simulink model "Joint_space_Traj"  (R2019b)
settings: Solver=FixedStepAuto  StartTime=0.0  StopTime=8  FixedStep=0.01  RelTol=1e-3
settings Model: Creator=gasserelazab  LastModifiedBy=gasserelazab

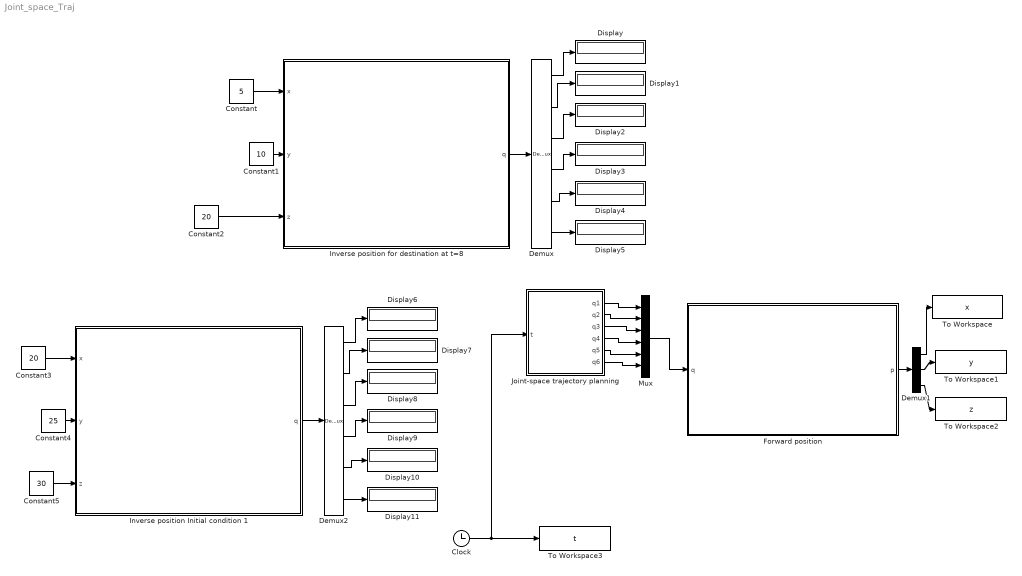
== system Joint_space_Traj ==
  Clock : Clock
  Constant : Constant  Value=5
  Constant1 : Constant  Value=10
  Constant2 : Constant  Value=20
  Constant3 : Constant  Value=20
  Constant4 : Constant  Value=25
  Constant5 : Constant  Value=30
  Demux : Demux  Outputs=6
  Demux1 : Demux  Outputs=3
  Demux2 : Demux  Outputs=6
  Display{,1..11} (12 alike) : Display
  "Forward position " : MATLAB Function  TreatAsAtomicUnit=on
  Inverse position Initial condition 1 : MATLAB Function  TreatAsAtomicUnit=on
  "Inverse position for destination at t=8 " : MATLAB Function  TreatAsAtomicUnit=on
  "Joint-space trajectory planning " : MATLAB Function  TreatAsAtomicUnit=on
  Mux : Mux  Inputs=6
  To Workspace : ToWorkspace  VariableName=x  SampleTime=-1
  To Workspace1 : ToWorkspace  VariableName=y  SampleTime=-1
  To Workspace2 : ToWorkspace  VariableName=z  SampleTime=-1
  To Workspace3 : ToWorkspace  VariableName=t  SampleTime=-1
  wires:
  Constant2/1 -> "Inverse position for destination at t=8 "/3(z)
  Constant1/1 -> "Inverse position for destination at t=8 "/2(y)
  Constant/1 -> "Inverse position for destination at t=8 "/1(x)
  "Inverse position for destination at t=8 "/1(q) -> Demux/1
  Demux/1 -> Display/1
  Demux/2 -> Display1/1
  Demux/3 -> Display2/1
  Demux/4 -> Display3/1
  Demux/5 -> Display4/1
  Demux/6 -> Display5/1
  Clock/1 -> To Workspace3/1, "Joint-space trajectory planning "/1(t)
  "Joint-space trajectory planning "/1(q1) -> Mux/1
  "Joint-space trajectory planning "/2(q2) -> Mux/2
  "Joint-space trajectory planning "/3(q3) -> Mux/3
  "Joint-space trajectory planning "/4(q4) -> Mux/4
  "Joint-space trajectory planning "/5(q5) -> Mux/5
  "Joint-space trajectory planning "/6(q6) -> Mux/6
  Mux/1 -> "Forward position "/1(q)
  "Forward position "/1(p) -> Demux1/1
  Demux1/1 -> To Workspace/1
  Demux1/2 -> To Workspace1/1
  Demux1/3 -> To Workspace2/1
  Demux2/4 -> Display9/1
  Inverse position Initial condition 1/1(q) -> Demux2/1
  Demux2/5 -> Display10/1
  Demux2/6 -> Display11/1
  Demux2/3 -> Display8/1
  Demux2/2 -> Display7/1
  Constant4/1 -> Inverse position Initial condition 1/2(y)
  Constant5/1 -> Inverse position Initial condition 1/3(z)
  Demux2/1 -> Display6/1
  Constant3/1 -> Inverse position Initial condition 1/1(x)

== matlab function Joint_space_Traj/Inverse position for destination at t=8  ==
  data: q output; x input; y input; z input
function q   = fcn(x, y, z)

qnew=[0;0;0;0;0;0];
qold=[50;50;50;50;50;50];

i=100;
dog=true;

while (i>0 && dog)
    q1=qold(1,1);
    q2=qold(2,1);
    q3=qold(3,1);
    q4=qold(4,1);
    q5=qold(5,1);
    q6=qold(6,1);
    
    F= [ 10*cos((pi*(q1 - 90))/180)*sin((pi*(q2 - 90))/180) - 10*sin((pi*(q5 + 90))/180)*(sin((pi*(q1 - 90))/180)*sin((pi*(q4 + 90))/180) - cos((pi*(q1 - 90))/180)*cos((pi*(q2 - 90))/180)*cos((pi*(q4 + 90))/180)) - x + cos((pi*(q1 - 90))/180)*sin((pi*(q2 - 90))/180)*(q3 + 10) - 10*cos((pi*(q1 - 90))/180)*cos((pi*(q5 + 90))/180)*sin((pi*(q2 - 90))/180);...
 10*sin((pi*(q5 + 90))/180)*(cos((pi*(q1 - 90))/180)*sin((pi*(q4 + 90))/180) + cos((pi*(q2 - 90))/180)*cos((pi*(q4 + 90))/180)*sin((pi*(q1 - 90))/180)) - y + 10*sin((pi*(q1 - 90))/180)*sin((pi*(q2 - 90))/180) + sin((pi*(q1 - 90))/180)*sin((pi*(q2 - 90))/180)*(q3 + 10) - 10*cos((pi*(q5 + 90))/180)*sin((pi*(q1 - 90))/180)*sin((pi*(q2 - 90))/180);...
                                                                                                                                                10*cos((pi*(q2 - 90))/180) - z + cos((pi*(q2 - 90))/180)*(q3 + 10) - 10*cos((pi*(q2 - 90))/180)*cos((pi*(q5 + 90))/180) - 10*cos((pi*(q4 + 90))/180)*sin((pi*(q2 - 90))/180)*sin((pi*(q5 + 90))/180) + 10];
 FJ= [ (pi*cos((pi*(q5 + 90))/180)*sin((pi*(q1 - 90))/180)*sin((pi*(q2 - 90))/180))/18 - (pi*sin((pi*(q1 - 90))/180)*sin((pi*(q2 - 90))/180))/18 - (pi*sin((pi*(q1 - 90))/180)*sin((pi*(q2 - 90))/180)*(q3 + 10))/180 - 10*sin((pi*(q5 + 90))/180)*((pi*cos((pi*(q1 - 90))/180)*sin((pi*(q4 + 90))/180))/180 + (pi*cos((pi*(q2 - 90))/180)*cos((pi*(q4 + 90))/180)*sin((pi*(q1 - 90))/180))/180), (pi*cos((pi*(q1 - 90))/180)*cos((pi*(q2 - 90))/180))/18 + (pi*cos((pi*(q1 - 90))/180)*cos((pi*(q2 - 90))/180)*(q3 + 10))/180 - (pi*cos((pi*(q1 - 90))/180)*cos((pi*(q2 - 90))/180)*cos((pi*(q5 + 90))/180))/18 - (pi*cos((pi*(q1 - 90))/180)*cos((pi*(q4 + 90))/180)*sin((pi*(q2 - 90))/180)*sin((pi*(q5 + 90))/180))/18, cos((pi*(q1 - 90))/180)*sin((pi*(q2 - 90))/180), -10*sin((pi*(q5 + 90))/180)*((pi*cos((pi*(q4 + 90))/180)*sin((pi*(q1 - 90))/180))/180 + (pi*cos((pi*(q1 - 90))/180)*cos((pi*(q2 - 90))/180)*sin((pi*(q4 + 90))/180))/180), (pi*cos((pi*(q1 - 90))/180)*sin((pi*(q2 - 90))/180)*sin((pi*(q5 + 90))/180))/18 - (pi*cos((pi*(q5 + 90))/180)*(sin((pi*(q1 - 90))/180)*sin((pi*(q4 + 90))/180) - cos((pi*(q1 - 90))/180)*cos((pi*(q2 - 90))/180)*cos((pi*(q4 + 90))/180)))/18, 0;...
 (pi*cos((pi*(q1 - 90))/180)*sin((pi*(q2 - 90))/180))/18 - 10*sin((pi*(q5 + 90))/180)*((pi*sin((pi*(q1 - 90))/180)*sin((pi*(q4 + 90))/180))/180 - (pi*cos((pi*(q1 - 90))/180)*cos((pi*(q2 - 90))/180)*cos((pi*(q4 + 90))/180))/180) + (pi*cos((pi*(q1 - 90))/180)*sin((pi*(q2 - 90))/180)*(q3 + 10))/180 - (pi*cos((pi*(q1 - 90))/180)*cos((pi*(q5 + 90))/180)*sin((pi*(q2 - 90))/180))/18, (pi*cos((pi*(q2 - 90))/180)*sin((pi*(q1 - 90))/180))/18 + (pi*cos((pi*(q2 - 90))/180)*sin((pi*(q1 - 90))/180)*(q3 + 10))/180 - (pi*cos((pi*(q2 - 90))/180)*cos((pi*(q5 + 90))/180)*sin((pi*(q1 - 90))/180))/18 - (pi*cos((pi*(q4 + 90))/180)*sin((pi*(q1 - 90))/180)*sin((pi*(q2 - 90))/180)*sin((pi*(q5 + 90))/180))/18, sin((pi*(q1 - 90))/180)*sin((pi*(q2 - 90))/180),  10*sin((pi*(q5 + 90))/180)*((pi*cos((pi*(q1 - 90))/180)*cos((pi*(q4 + 90))/180))/180 - (pi*cos((pi*(q2 - 90))/180)*sin((pi*(q1 - 90))/180)*sin((pi*(q4 + 90))/180))/180), (pi*cos((pi*(q5 + 90))/180)*(cos((pi*(q1 - 90))/180)*sin((pi*(q4 + 90))/180) + cos((pi*(q2 - 90))/180)*cos((pi*(q4 + 90))/180)*sin((pi*(q1 - 90))/180)))/18 + (pi*sin((pi*(q1 - 90))/180)*sin((pi*(q2 - 90))/180)*sin((pi*(q5 + 90))/180))/18, 0;...
                                                                                                                                                                                                                                                                                                                                                                                         0,                                                                                                 (pi*cos((pi*(q5 + 90))/180)*sin((pi*(q2 - 90))/180))/18 - (pi*sin((pi*(q2 - 90))/180)*(q3 + 10))/180 - (pi*sin((pi*(q2 - 90))/180))/18 - (pi*cos((pi*(q2 - 90))/180)*cos((pi*(q4 + 90))/180)*sin((pi*(q5 + 90))/180))/18,                         cos((pi*(q2 - 90))/180),                                                                                           (pi*sin((pi*(q2 - 90))/180)*sin((pi*(q4 + 90))/180)*sin((pi*(q5 + 90))/180))/18,                                                                                                     (pi*cos((pi*(q2 - 90))/180)*sin((pi*(q5 + 90))/180))/18 - (pi*cos((pi*(q4 + 90))/180)*cos((pi*(q5 + 90))/180)*sin((pi*(q2 - 90))/180))/18, 0];
 

    inverseFJ= transpose(FJ)*(inv(FJ*transpose(FJ)));
        
 
    qnew=qold-inverseFJ*F;
    %disp(inverseFJ*F);
    
  
   
    count=0;
   
   	for xx = 1:6
        if  ((qnew(xx,1)-qold(xx,1)<0.1) && (qnew(xx,1)-qold(xx,1)>-0.1 ))       
             count=count+1;
         end
   
    end
    
    if( count == 6)
        dog=false;
    end
    
    i=i-1;
    
    %disp(i);
    
    qold=qnew;
    
end
q=qold;

== matlab function Joint_space_Traj/Joint-space trajectory planning  ==
  data: t input; q1 output; q2 output; q3 output; q4 output; q5 output; q6 output
function [q1,q2,q3,q4,q5,q6] = fcn(t)

q1= -21.89 + 1.75125*t^(2) - 0.146*t^(3);
q2= 38.51 + 1.415*t^(2) -0.118*t^(3);
q3= 14.89 + -1.30125*t^(2) + 0.1084375*t^(3);
q4= 20.75 + 0.3740526*t^(2) - 0.031171875*t^(3);
q5= 8.891 + 1.0542*t^(2) - 0.0878*t^(3);
q6=0;

== matlab function Joint_space_Traj/Forward position  ==
  data: p output; q input
function p  = fcn(q)
q1= q(1);
q2= q(2);
q3= q(3);
q4= q(4);
q5= q(5);
q6= q(6);
L1=10;
L2=10;
L3=10;
L4=10;
pp= [ sin((pi*q6)/180)*(cos((pi*(q4 + 90))/180)*sin((pi*(q1 - 90))/180) + cos((pi*(q1 - 90))/180)*cos((pi*(q2 - 90))/180)*sin((pi*(q4 + 90))/180)) - cos((pi*q6)/180)*(cos((pi*(q5 + 90))/180)*(sin((pi*(q1 - 90))/180)*sin((pi*(q4 + 90))/180) - cos((pi*(q1 - 90))/180)*cos((pi*(q2 - 90))/180)*cos((pi*(q4 + 90))/180)) - cos((pi*(q1 - 90))/180)*sin((pi*(q2 - 90))/180)*sin((pi*(q5 + 90))/180)),   sin((pi*q6)/180)*(cos((pi*(q5 + 90))/180)*(sin((pi*(q1 - 90))/180)*sin((pi*(q4 + 90))/180) - cos((pi*(q1 - 90))/180)*cos((pi*(q2 - 90))/180)*cos((pi*(q4 + 90))/180)) - cos((pi*(q1 - 90))/180)*sin((pi*(q2 - 90))/180)*sin((pi*(q5 + 90))/180)) + cos((pi*q6)/180)*(cos((pi*(q4 + 90))/180)*sin((pi*(q1 - 90))/180) + cos((pi*(q1 - 90))/180)*cos((pi*(q2 - 90))/180)*sin((pi*(q4 + 90))/180)), - sin((pi*(q5 + 90))/180)*(sin((pi*(q1 - 90))/180)*sin((pi*(q4 + 90))/180) - cos((pi*(q1 - 90))/180)*cos((pi*(q2 - 90))/180)*cos((pi*(q4 + 90))/180)) - cos((pi*(q1 - 90))/180)*cos((pi*(q5 + 90))/180)*sin((pi*(q2 - 90))/180), cos((pi*(q1 - 90))/180)*sin((pi*(q2 - 90))/180)*(L2 + q3) - L4*(sin((pi*(q5 + 90))/180)*(sin((pi*(q1 - 90))/180)*sin((pi*(q4 + 90))/180) - cos((pi*(q1 - 90))/180)*cos((pi*(q2 - 90))/180)*cos((pi*(q4 + 90))/180)) + cos((pi*(q1 - 90))/180)*cos((pi*(q5 + 90))/180)*sin((pi*(q2 - 90))/180)) + L3*cos((pi*(q1 - 90))/180)*sin((pi*(q2 - 90))/180);
 cos((pi*q6)/180)*(cos((pi*(q5 + 90))/180)*(cos((pi*(q1 - 90))/180)*sin((pi*(q4 + 90))/180) + cos((pi*(q2 - 90))/180)*cos((pi*(q4 + 90))/180)*sin((pi*(q1 - 90))/180)) + sin((pi*(q1 - 90))/180)*sin((pi*(q2 - 90))/180)*sin((pi*(q5 + 90))/180)) - sin((pi*q6)/180)*(cos((pi*(q1 - 90))/180)*cos((pi*(q4 + 90))/180) - cos((pi*(q2 - 90))/180)*sin((pi*(q1 - 90))/180)*sin((pi*(q4 + 90))/180)), - sin((pi*q6)/180)*(cos((pi*(q5 + 90))/180)*(cos((pi*(q1 - 90))/180)*sin((pi*(q4 + 90))/180) + cos((pi*(q2 - 90))/180)*cos((pi*(q4 + 90))/180)*sin((pi*(q1 - 90))/180)) + sin((pi*(q1 - 90))/180)*sin((pi*(q2 - 90))/180)*sin((pi*(q5 + 90))/180)) - cos((pi*q6)/180)*(cos((pi*(q1 - 90))/180)*cos((pi*(q4 + 90))/180) - cos((pi*(q2 - 90))/180)*sin((pi*(q1 - 90))/180)*sin((pi*(q4 + 90))/180)),   sin((pi*(q5 + 90))/180)*(cos((pi*(q1 - 90))/180)*sin((pi*(q4 + 90))/180) + cos((pi*(q2 - 90))/180)*cos((pi*(q4 + 90))/180)*sin((pi*(q1 - 90))/180)) - cos((pi*(q5 + 90))/180)*sin((pi*(q1 - 90))/180)*sin((pi*(q2 - 90))/180), L4*(sin((pi*(q5 + 90))/180)*(cos((pi*(q1 - 90))/180)*sin((pi*(q4 + 90))/180) + cos((pi*(q2 - 90))/180)*cos((pi*(q4 + 90))/180)*sin((pi*(q1 - 90))/180)) - cos((pi*(q5 + 90))/180)*sin((pi*(q1 - 90))/180)*sin((pi*(q2 - 90))/180)) + sin((pi*(q1 - 90))/180)*sin((pi*(q2 - 90))/180)*(L2 + q3) + L3*sin((pi*(q1 - 90))/180)*sin((pi*(q2 - 90))/180);
                                                                                                                                                                                 cos((pi*q6)/180)*(cos((pi*(q2 - 90))/180)*sin((pi*(q5 + 90))/180) - cos((pi*(q4 + 90))/180)*cos((pi*(q5 + 90))/180)*sin((pi*(q2 - 90))/180)) - sin((pi*q6)/180)*sin((pi*(q2 - 90))/180)*sin((pi*(q4 + 90))/180),                                                                                                                                                                                 - sin((pi*q6)/180)*(cos((pi*(q2 - 90))/180)*sin((pi*(q5 + 90))/180) - cos((pi*(q4 + 90))/180)*cos((pi*(q5 + 90))/180)*sin((pi*(q2 - 90))/180)) - cos((pi*q6)/180)*sin((pi*(q2 - 90))/180)*sin((pi*(q4 + 90))/180),                                                                                                     - cos((pi*(q2 - 90))/180)*cos((pi*(q5 + 90))/180) - cos((pi*(q4 + 90))/180)*sin((pi*(q2 - 90))/180)*sin((pi*(q5 + 90))/180),                                                                                                                                                L1 - L4*(cos((pi*(q2 - 90))/180)*cos((pi*(q5 + 90))/180) + cos((pi*(q4 + 90))/180)*sin((pi*(q2 - 90))/180)*sin((pi*(q5 + 90))/180)) + cos((pi*(q2 - 90))/180)*(L2 + q3) + L3*cos((pi*(q2 - 90))/180);
                                                                                                                                                                                                                                                                                                                                                                                               0,                                                                                                                                                                                                                                                                                                                                                                                                 0,                                                                                                                                                                                                                               0,                                                                                                                                                                                                                                                                                                                                                   1];
x=pp(1,4);
y=pp(2,4);
z=pp(3,4);
p= [x;y;z];

== matlab function Joint_space_Traj/Inverse position Initial condition 1 ==
  data: q output; x input; y input; z input
function q   = fcn(x, y, z)

qnew=[0;0;0;0;0;0];
qold=[50;50;50;50;50;50];

i=100;
dog=true;

while (i>0 && dog)
    q1=qold(1,1);
    q2=qold(2,1);
    q3=qold(3,1);
    q4=qold(4,1);
    q5=qold(5,1);
    q6=qold(6,1);
    
    F= [ 10*cos((pi*(q1 - 90))/180)*sin((pi*(q2 - 90))/180) - 10*sin((pi*(q5 + 90))/180)*(sin((pi*(q1 - 90))/180)*sin((pi*(q4 + 90))/180) - cos((pi*(q1 - 90))/180)*cos((pi*(q2 - 90))/180)*cos((pi*(q4 + 90))/180)) - x + cos((pi*(q1 - 90))/180)*sin((pi*(q2 - 90))/180)*(q3 + 10) - 10*cos((pi*(q1 - 90))/180)*cos((pi*(q5 + 90))/180)*sin((pi*(q2 - 90))/180);...
 10*sin((pi*(q5 + 90))/180)*(cos((pi*(q1 - 90))/180)*sin((pi*(q4 + 90))/180) + cos((pi*(q2 - 90))/180)*cos((pi*(q4 + 90))/180)*sin((pi*(q1 - 90))/180)) - y + 10*sin((pi*(q1 - 90))/180)*sin((pi*(q2 - 90))/180) + sin((pi*(q1 - 90))/180)*sin((pi*(q2 - 90))/180)*(q3 + 10) - 10*cos((pi*(q5 + 90))/180)*sin((pi*(q1 - 90))/180)*sin((pi*(q2 - 90))/180);...
                                                                                                                                                10*cos((pi*(q2 - 90))/180) - z + cos((pi*(q2 - 90))/180)*(q3 + 10) - 10*cos((pi*(q2 - 90))/180)*cos((pi*(q5 + 90))/180) - 10*cos((pi*(q4 + 90))/180)*sin((pi*(q2 - 90))/180)*sin((pi*(q5 + 90))/180) + 10];
 FJ= [ (pi*cos((pi*(q5 + 90))/180)*sin((pi*(q1 - 90))/180)*sin((pi*(q2 - 90))/180))/18 - (pi*sin((pi*(q1 - 90))/180)*sin((pi*(q2 - 90))/180))/18 - (pi*sin((pi*(q1 - 90))/180)*sin((pi*(q2 - 90))/180)*(q3 + 10))/180 - 10*sin((pi*(q5 + 90))/180)*((pi*cos((pi*(q1 - 90))/180)*sin((pi*(q4 + 90))/180))/180 + (pi*cos((pi*(q2 - 90))/180)*cos((pi*(q4 + 90))/180)*sin((pi*(q1 - 90))/180))/180), (pi*cos((pi*(q1 - 90))/180)*cos((pi*(q2 - 90))/180))/18 + (pi*cos((pi*(q1 - 90))/180)*cos((pi*(q2 - 90))/180)*(q3 + 10))/180 - (pi*cos((pi*(q1 - 90))/180)*cos((pi*(q2 - 90))/180)*cos((pi*(q5 + 90))/180))/18 - (pi*cos((pi*(q1 - 90))/180)*cos((pi*(q4 + 90))/180)*sin((pi*(q2 - 90))/180)*sin((pi*(q5 + 90))/180))/18, cos((pi*(q1 - 90))/180)*sin((pi*(q2 - 90))/180), -10*sin((pi*(q5 + 90))/180)*((pi*cos((pi*(q4 + 90))/180)*sin((pi*(q1 - 90))/180))/180 + (pi*cos((pi*(q1 - 90))/180)*cos((pi*(q2 - 90))/180)*sin((pi*(q4 + 90))/180))/180), (pi*cos((pi*(q1 - 90))/180)*sin((pi*(q2 - 90))/180)*sin((pi*(q5 + 90))/180))/18 - (pi*cos((pi*(q5 + 90))/180)*(sin((pi*(q1 - 90))/180)*sin((pi*(q4 + 90))/180) - cos((pi*(q1 - 90))/180)*cos((pi*(q2 - 90))/180)*cos((pi*(q4 + 90))/180)))/18, 0;...
 (pi*cos((pi*(q1 - 90))/180)*sin((pi*(q2 - 90))/180))/18 - 10*sin((pi*(q5 + 90))/180)*((pi*sin((pi*(q1 - 90))/180)*sin((pi*(q4 + 90))/180))/180 - (pi*cos((pi*(q1 - 90))/180)*cos((pi*(q2 - 90))/180)*cos((pi*(q4 + 90))/180))/180) + (pi*cos((pi*(q1 - 90))/180)*sin((pi*(q2 - 90))/180)*(q3 + 10))/180 - (pi*cos((pi*(q1 - 90))/180)*cos((pi*(q5 + 90))/180)*sin((pi*(q2 - 90))/180))/18, (pi*cos((pi*(q2 - 90))/180)*sin((pi*(q1 - 90))/180))/18 + (pi*cos((pi*(q2 - 90))/180)*sin((pi*(q1 - 90))/180)*(q3 + 10))/180 - (pi*cos((pi*(q2 - 90))/180)*cos((pi*(q5 + 90))/180)*sin((pi*(q1 - 90))/180))/18 - (pi*cos((pi*(q4 + 90))/180)*sin((pi*(q1 - 90))/180)*sin((pi*(q2 - 90))/180)*sin((pi*(q5 + 90))/180))/18, sin((pi*(q1 - 90))/180)*sin((pi*(q2 - 90))/180),  10*sin((pi*(q5 + 90))/180)*((pi*cos((pi*(q1 - 90))/180)*cos((pi*(q4 + 90))/180))/180 - (pi*cos((pi*(q2 - 90))/180)*sin((pi*(q1 - 90))/180)*sin((pi*(q4 + 90))/180))/180), (pi*cos((pi*(q5 + 90))/180)*(cos((pi*(q1 - 90))/180)*sin((pi*(q4 + 90))/180) + cos((pi*(q2 - 90))/180)*cos((pi*(q4 + 90))/180)*sin((pi*(q1 - 90))/180)))/18 + (pi*sin((pi*(q1 - 90))/180)*sin((pi*(q2 - 90))/180)*sin((pi*(q5 + 90))/180))/18, 0;...
                                                                                                                                                                                                                                                                                                                                                                                         0,                                                                                                 (pi*cos((pi*(q5 + 90))/180)*sin((pi*(q2 - 90))/180))/18 - (pi*sin((pi*(q2 - 90))/180)*(q3 + 10))/180 - (pi*sin((pi*(q2 - 90))/180))/18 - (pi*cos((pi*(q2 - 90))/180)*cos((pi*(q4 + 90))/180)*sin((pi*(q5 + 90))/180))/18,                         cos((pi*(q2 - 90))/180),                                                                                           (pi*sin((pi*(q2 - 90))/180)*sin((pi*(q4 + 90))/180)*sin((pi*(q5 + 90))/180))/18,                                                                                                     (pi*cos((pi*(q2 - 90))/180)*sin((pi*(q5 + 90))/180))/18 - (pi*cos((pi*(q4 + 90))/180)*cos((pi*(q5 + 90))/180)*sin((pi*(q2 - 90))/180))/18, 0];
 

    inverseFJ= transpose(FJ)*(inv(FJ*transpose(FJ)));
        
 
    qnew=qold-inverseFJ*F;
    %disp(inverseFJ*F);
    
  
   
    count=0;
   
   	for xx = 1:6
        if  ((qnew(xx,1)-qold(xx,1)<0.1) && (qnew(xx,1)-qold(xx,1)>-0.1 ))       
             count=count+1;
         end
   
    end
    
    if( count == 6)
        dog=false;
    end
    
    i=i-1;
    
    %disp(i);
    
    qold=qnew;
    
end
q=qold;
